simulink model "simulator"  (R2018b)
settings: Solver=VariableStepAuto  StartTime=0.0  StopTime=21  RelTol=1e-3  EnableMultiTasking=on
values from neighbouring files (symbols this model uses):
  acc_seed = randi(1000, [3, 1])    [init.m]
  anchors = [-4.715, -4.539, 2.67 ... (first row only)    [init.m]
  bias = [0.02998003, -0.03306038,  0.05456951 ... (first row only)    [init.m]
  gyro_seed = randi(1000, [3, 1])    [init.m]
  h = 0.002    [init.m]
  k = 2.2e-8    (= 2.2e-08)    [init_quadcopter_model.m]
  omega_max_lim = 2500    [init_inner_PD_d.m]
  omega_min_lim = 0    [init_inner_PD_d.m]
  outlier_seed = randi(1000, [4, 1])    [init.m]
  P_init = diag([10000,10000,1,0.0001,0.0001,0.0001,0.0001,0.0001,0.0001])    [init.m]
  PosD = 0.24    [init.m]
  PosI = 0    [init.m]
  PosP = 0.20    (= 0.2)    [init.m]
  procent_modifier = 1.96    [init.m]
  Q = diag([4.8366*h*h 4.8366*h*h 0.4530*h*h 4.8366*h 4.8366*h 0.4530*h 0.0083*h 0.0083*h 0.0547*h].^2)    [init.m]
  q_init = [1; 0; 0; 0]    [init.m]
  R = [R_alti R_uwb]    [init.m]
  Rotmat_init = eye(3)    [init.m]
  uwb_seed = randi(1000, [4, 1])    [init.m]
  uwb_var = 0.0625    [init.m]
  x_hat_init = [0; 0; 0; 0; 0; 0; 0; 0; 0]    [init.m]
  yaw_seed = randi(1000, 1)    [init.m]
undefined symbols (not defined in the file or in its folder): sigbuilder_block
libraries: commchan3 x17, simulink x2, dspinverses x1, dspmtrx3 x1
settings Model: Creator=Daniel  LastModifiedBy=sstroobants
settings DataIOCC: LimitDataPoints=on
settings OptimizationCC: LifeSpan=inf
settings DebuggingCC: AllowSymbolicDim=off  SFUnexpectedBacktrackingDiag=warning  SFNoUnconditionalDefaultTransitionDiag=warning  UnderSpecifiedDimensionMsg=warning
settings ModelReferenceCC: PropagateSignalLabelsOutOfModel=off
settings SFSimCC: SimUseLocalCustomCode=off
settings RTWCC: RTWUseLocalCustomCode=off
settings CodeAppCC: StateflowObjectComments=on
settings GRTTargetCC: TargetLangStandard=C89/C90 (ANSI)
settings ConfigComp: CovMetricSettings=dw  CovHtmlReporting=on  CovSaveCumulativeToWorkspaceVar=on  CovSaveSingleToWorkspaceVar=on  CovExternalEMLEnable=off

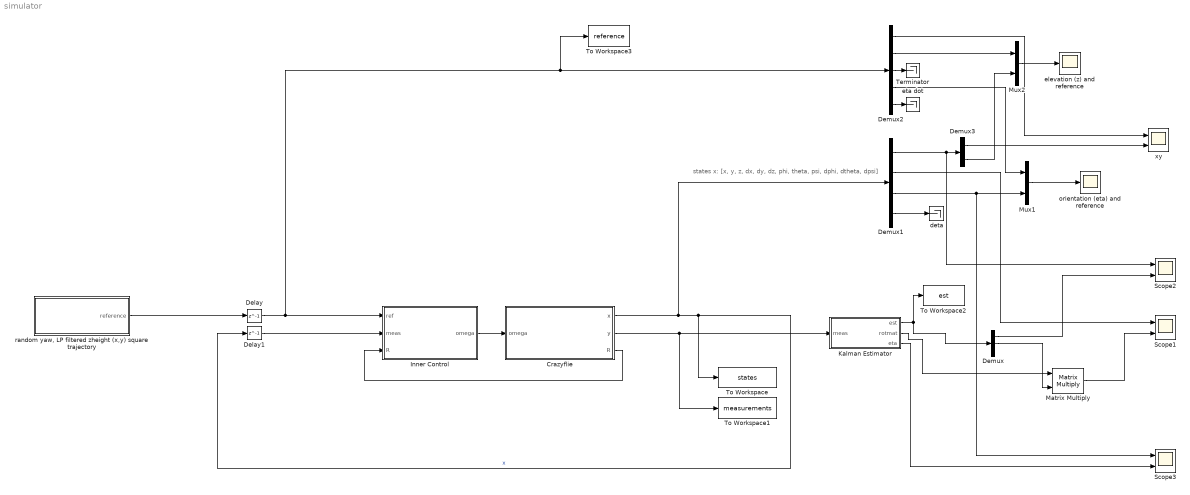
== system simulator ==
  note: states x: [x, y, z, dx, dy, dz, phi, theta, psi, dphi, dtheta, dpsi]
  "   deta" : Terminator
  "   eta dot" : Terminator
  Crazyflie : Subsystem
  Delay : Delay  DelayLength=1  InitialCondition=0  SampleTime=0.002
  Delay1 : Delay  DelayLength=1  InitialCondition=0  SampleTime=0.002
  Demux : Demux  Outputs=3
  Demux1 : Demux  Outputs=[3,3,3,3]
  Demux2 : Demux  Outputs=[2,1,3,3,3]
  Demux3 : Demux  Outputs=[2,1]
  Inner Control : Subsystem
  Kalman Estimator : Subsystem
  Matrix Multiply : Product  Multiplication=Matrix(*)
  Mux1 : Mux  Inputs=2
  Mux2 : Mux  Inputs=2
  Scope1 : Scope  NumInputPorts=2
  Scope2 : Scope  NumInputPorts=2
  Scope3 : Scope  NumInputPorts=2
  Terminator : Terminator
  To Workspace : ToWorkspace  VariableName=states  SaveFormat=Timeseries  SampleTime=-1
  To Workspace1 : ToWorkspace  VariableName=measurements  SaveFormat=Timeseries  SampleTime=-1
  To Workspace2 : ToWorkspace  VariableName=est  SaveFormat=Timeseries  SampleTime=-1
  To Workspace3 : ToWorkspace  VariableName=reference  SaveFormat=Timeseries  SampleTime=-1
  elevation (z) and reference : Scope
  orientation (eta) and reference : Scope
  "random yaw, LP filtered zheight (x,y) square trajectory " : Subsystem
  xy : Scope  NumInputPorts=2
  wires:
  Mux2/1 -> elevation (z) and reference/1
  Mux1/1 -> orientation (eta) and reference/1
  Demux2/5 -> "   eta dot"/1
  Demux2/1 -> xy/1
  Demux1/1 -> Demux3/1, Scope2/1
  Delay/1 -> To Workspace3/1, Demux2/1, Inner Control/1(ref)
  Delay1/1 -> Inner Control/2(meas)
  Demux1/4 -> "   deta"/1
  Demux3/1 -> xy/2
  "random yaw, LP filtered zheight (x,y) square trajectory "/1(reference) -> Delay/1
  Demux2/2 -> Mux2/1
  Demux3/2 -> Mux2/2
  Demux1/3 -> Scope3/1, Mux1/2
  Demux2/4 -> Mux1/1
  Inner Control/1(omega) -> Crazyflie/1(omega)
  Crazyflie/1(x) -> To Workspace/1, Delay1/1, Demux1/1  "x"
  Crazyflie/2(y) -> To Workspace1/1, Kalman Estimator/1(meas)
  Kalman Estimator/1(est) -> Demux/1, To Workspace2/1
  Demux/2 -> Matrix Multiply/2
  Demux1/2 -> Scope1/1
  Matrix Multiply/1 -> Scope1/2
  Kalman Estimator/2(rotmat) -> Matrix Multiply/1
  Demux/1 -> Scope2/2
  Kalman Estimator/3(eta) -> Scope3/2
  Crazyflie/3(R) -> Inner Control/3(R)
  Demux2/3 -> Terminator/1

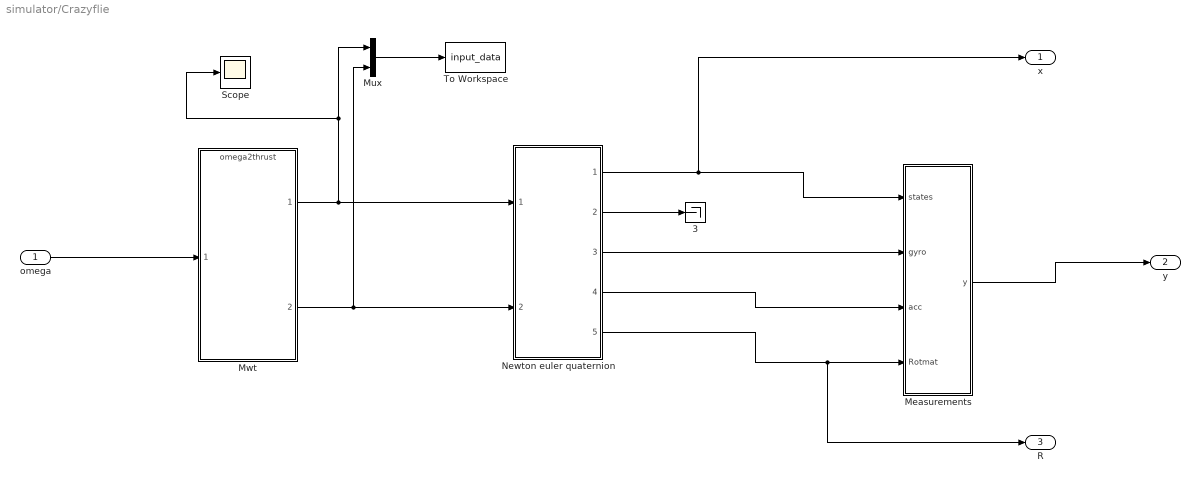
== system simulator/Crazyflie ==
  omega : Inport
  "   3" : Terminator
  Measurements : Subsystem
  Mux : Mux  Inputs=2
  Mwt : ModelReference  ModelNameDialog=omega2thrust.mdl  SimulationMode=Normal  ModelReferenceVersion=1.5
  Newton euler quaternion : ModelReference  ModelNameDialog=quadcopter_model_c_NewtonEuler.mdl  SimulationMode=Normal  ModelReferenceVersion=1.346
  Scope : Scope
  To Workspace : ToWorkspace  VariableName=input_data  SaveFormat=Timeseries  SampleTime=-1
  x : Outport
  y : Outport  Port=2
  R : Outport  Port=3
  wires:
  Newton euler quaternion/2 -> "   3"/1
  Newton euler quaternion/5 -> R/1, Measurements/4(Rotmat)
  Mwt/1 -> Mux/1, Scope/1, Newton euler quaternion/1
  omega/1 -> Mwt/1
  Newton euler quaternion/1 -> x/1, Measurements/1(states)
  Mwt/2 -> Mux/2, Newton euler quaternion/2
  Newton euler quaternion/3 -> Measurements/2(gyro)
  Newton euler quaternion/4 -> Measurements/3(acc)
  Measurements/1(y) -> y/1
  Mux/1 -> To Workspace/1

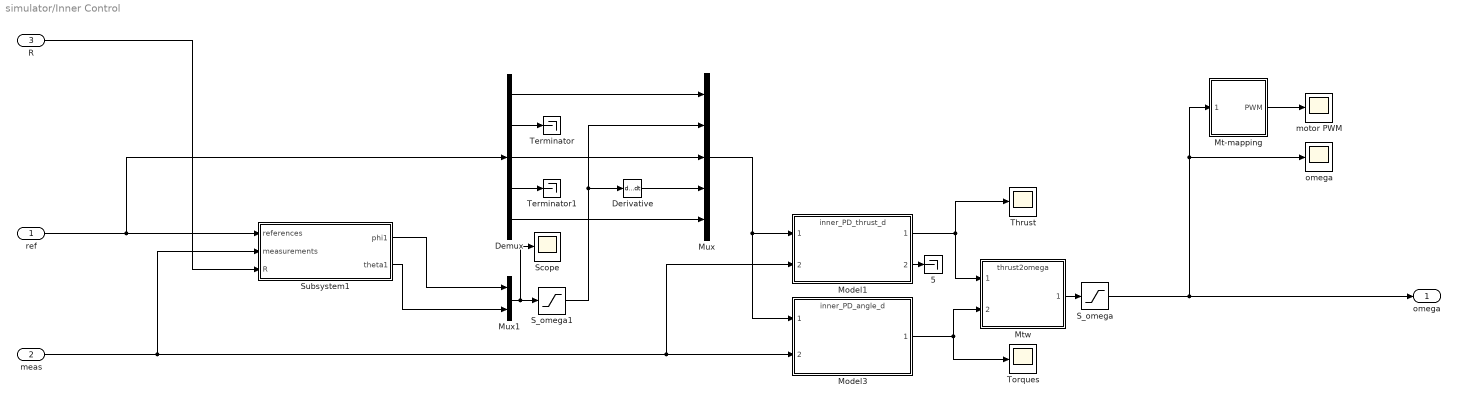
== system simulator/Inner Control ==
  ref : Inport
  meas : Inport  Port=2
  R : Inport  Port=3
  "   5" : Terminator
  Demux : Demux  Outputs=[6,2,1,2,1]
  Derivative : Derivative
  Model1 : ModelReference  ModelNameDialog=inner_PD_thrust_d.slx  SimulationMode=Normal  ModelReferenceVersion=1.83
  Model3 : ModelReference  ModelNameDialog=inner_PD_angle_d.slx  SimulationMode=Normal  ModelReferenceVersion=1.87
  Mt-mapping : Subsystem
  Mtw : ModelReference  ModelNameDialog=thrust2omega.mdl  SimulationMode=Normal  ModelReferenceVersion=1.5
  Mux : Mux  Inputs=[6,2,1,2,1]
  Mux1 : Mux  Inputs=2
  S_omega : Saturate  UpperLimit=omega_max_lim  LowerLimit=omega_min_lim
  S_omega1 : Saturate
  Scope : Scope
  Subsystem1 : Subsystem
  Terminator : Terminator
  Terminator1 : Terminator
  Thrust : Scope
  Torques : Scope
  motor PWM : Scope
  "omega " : Scope
  omega : Outport
  wires:
  Model1/2 -> "   5"/1
  Model3/1 -> Torques/1, Mtw/2
  Model1/1 -> Thrust/1, Mtw/1
  Mtw/1 -> S_omega/1
  S_omega/1 -> omega/1, Mt-mapping/1(omega), "omega "/1
  Mt-mapping/1(PWM) -> motor PWM/1
  ref/1 -> Subsystem1/1(references), Demux/1
  meas/1 -> Subsystem1/2(measurements), Model1/2, Model3/2
  Demux/1 -> Mux/1
  Mux1/1 -> Scope/1, S_omega1/1
  Derivative/1 -> Mux/4
  Demux/2 -> Terminator/1
  Demux/4 -> Terminator1/1
  Demux/3 -> Mux/3
  Demux/5 -> Mux/5
  Mux/1 -> Model3/1, Model1/1
  S_omega1/1 -> Derivative/1, Mux/2
  R/1 -> Subsystem1/3(R)
  Subsystem1/1(phi1) -> Mux1/1
  Subsystem1/2(theta1) -> Mux1/2

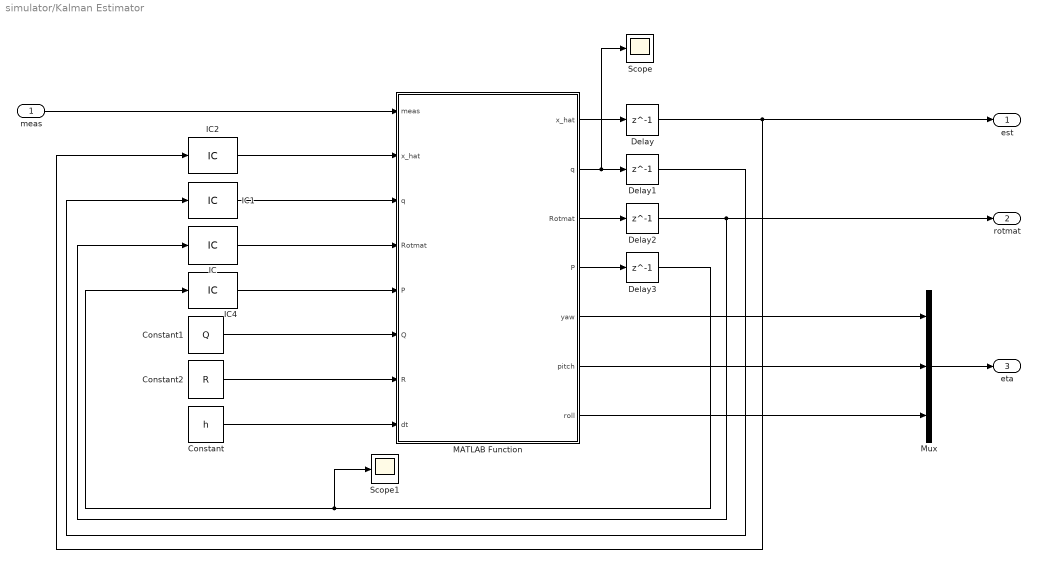
== system simulator/Kalman Estimator ==
  meas : Inport  PortDimensions=17
  Constant : Constant  Value=h
  Constant1 : Constant  Value=Q
  Constant2 : Constant  Value=R
  Delay{,1..3} (4 alike) : Delay  DelayLength=1
  IC : InitialCondition  Value=Rotmat_init
  IC1 : InitialCondition  Value=q_init
  IC2 : InitialCondition  Value=x_hat_init
  IC4 : InitialCondition  Value=P_init
  MATLAB Function : MATLAB Function  TreatAsAtomicUnit=on
  Mux : Mux  Inputs=3
  Scope : Scope
  Scope1 : Scope
  est : Outport  PortDimensions=9
  rotmat : Outport  Port=2  PortDimensions=[3 3]
  eta : Outport  Port=3  PortDimensions=3
  wires:
  meas/1 -> MATLAB Function/1(meas)
  Constant1/1 -> MATLAB Function/6(Q)
  IC/1 -> MATLAB Function/4("Rotmat ")
  IC1/1 -> MATLAB Function/3("q ")
  IC2/1 -> MATLAB Function/2("x_hat ")
  IC4/1 -> MATLAB Function/5("P ")
  MATLAB Function/1(x_hat) -> Delay/1
  MATLAB Function/2(q) -> Scope/1, Delay1/1
  MATLAB Function/3(Rotmat) -> Delay2/1
  MATLAB Function/4(P) -> Delay3/1
  Delay/1 -> est/1, IC2/1
  Delay1/1 -> IC1/1
  Delay2/1 -> IC/1, rotmat/1
  Delay3/1 -> Scope1/1, IC4/1
  Constant2/1 -> MATLAB Function/7(R)
  MATLAB Function/5(yaw) -> Mux/1
  MATLAB Function/6(pitch) -> Mux/2
  MATLAB Function/7(roll) -> Mux/3
  Mux/1 -> eta/1
  Constant/1 -> MATLAB Function/8(dt)

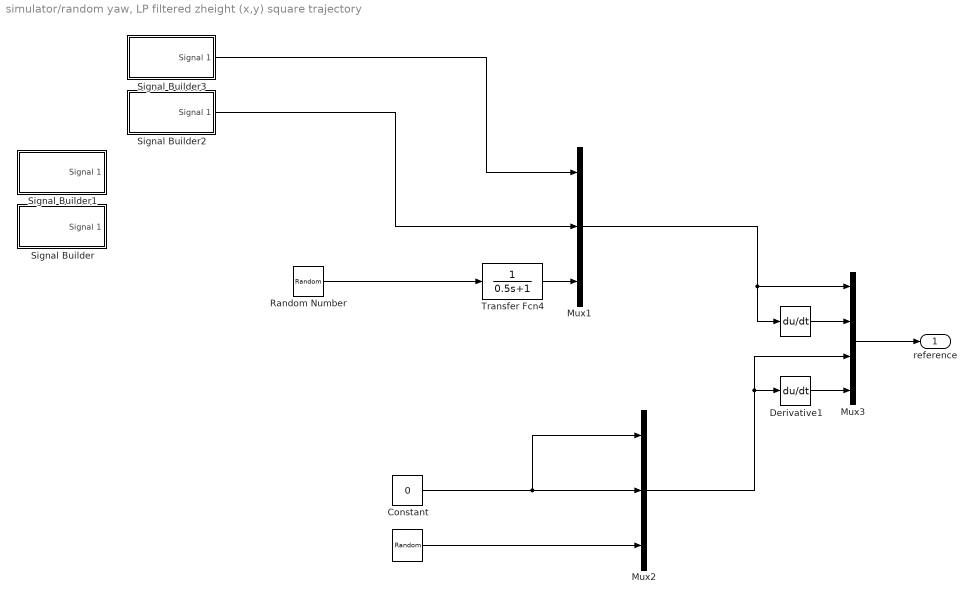
== system simulator/random yaw, LP filtered zheight (x,y) square trajectory  ==
  "   " : UniformRandomNumber  Minimum=-0.3  Maximum=0.3  Seed=yaw_seed  SampleTime=3
  "        " : Derivative
  Constant : Constant  Value=0
  Derivative1 : Derivative
  Mux1 : Mux  Inputs=3
  Mux2 : Mux  Inputs=3
  Mux3 : Mux  Inputs=[3,3,3,3]
  Random Number : RandomNumber  Mean=1.5  Variance=0.6  SampleTime=0.1
  Signal Builder : Subsystem  Tag=STV Subsys  LoadFcn=sigbuilder_block('load');  StartFcn=sigbuilder_block('start');  StopFcn=sigbuilder_block('stop');  ClipboardFcn=sigbuilder_block('clipboard');  mask(Sigbuilder block){tuvar=[0:10]}
      mask help: Simulink:masks:SigbuilderBlock_MD
      mask init:
      | if ~strcmp(get_param(bdroot(gcbh),'SimulationStatus'),'stopped') tuvar = sigbuilder_block('maskInit'); end
      settings: CopyFcn=sigbuilder_block('copy');  DeleteFcn=sigbuilder_block('delete');  ModelCloseFcn=sigbuilder_block('modelClose');  PreSaveFcn=sigbuilder_block('preSave');  PauseFcn=sigbuilder_block('pause');  ContinueFcn=sigbuilder_block('continue');  NameChangeFcn=sigbuilder_block('namechange');  OpenFcn=sigbuilder_block('open',[411 173.25 603 399.75 ]);  CloseFcn=sigbuilder_block('close');
      mask Display: plot(0, 0, 100, 100,[2, 2, 32, 32, 2], [68, 8, 8, 68, 68],[32, 2], [38, 38], [32, 19, 2],[53, 60, 44], [32, 17, 17, 2],[16, 16, 31, 31]);txt = getActiveGroup(gcbh);text(2, 100, txt,'verticalAlignment', 'top');
  Signal Builder1 : Subsystem  Tag=STV Subsys  LoadFcn=sigbuilder_block('load');  StartFcn=sigbuilder_block('start');  StopFcn=sigbuilder_block('stop');  ClipboardFcn=sigbuilder_block('clipboard');  mask(Sigbuilder block){tuvar=[0:10]}
      mask help: Simulink:masks:SigbuilderBlock_MD
      mask init:
      | if ~strcmp(get_param(bdroot(gcbh),'SimulationStatus'),'stopped') tuvar = sigbuilder_block('maskInit'); end
      settings: CopyFcn=sigbuilder_block('copy');  DeleteFcn=sigbuilder_block('delete');  ModelCloseFcn=sigbuilder_block('modelClose');  PreSaveFcn=sigbuilder_block('preSave');  PauseFcn=sigbuilder_block('pause');  ContinueFcn=sigbuilder_block('continue');  NameChangeFcn=sigbuilder_block('namechange');  OpenFcn=sigbuilder_block('open',[411 173.25 603 399.75 ]);  CloseFcn=sigbuilder_block('close');
      mask Display: plot(0, 0, 100, 100,[2, 2, 32, 32, 2], [68, 8, 8, 68, 68],[32, 2], [38, 38], [32, 19, 2],[53, 60, 44], [32, 17, 17, 2],[16, 16, 31, 31]);txt = getActiveGroup(gcbh);text(2, 100, txt,'verticalAlignment', 'top');
  Signal Builder2 : Subsystem  Tag=STV Subsys  LoadFcn=sigbuilder_block('load');  StartFcn=sigbuilder_block('start');  StopFcn=sigbuilder_block('stop');  ClipboardFcn=sigbuilder_block('clipboard');  mask(Sigbuilder block){tuvar=[0:10]}
      mask help: Simulink:masks:SigbuilderBlock_MD
      mask init:
      | if ~strcmp(get_param(bdroot(gcbh),'SimulationStatus'),'stopped') tuvar = sigbuilder_block('maskInit'); end
      settings: CopyFcn=sigbuilder_block('copy');  DeleteFcn=sigbuilder_block('delete');  ModelCloseFcn=sigbuilder_block('modelClose');  PreSaveFcn=sigbuilder_block('preSave');  PauseFcn=sigbuilder_block('pause');  ContinueFcn=sigbuilder_block('continue');  NameChangeFcn=sigbuilder_block('namechange');  OpenFcn=sigbuilder_block('open',[406.5 170.25 603 399.75 ]);  CloseFcn=sigbuilder_block('close');
      mask Display: plot(0, 0, 100, 100,[2, 2, 32, 32, 2], [68, 8, 8, 68, 68],[32, 2], [38, 38], [32, 19, 2],[53, 60, 44], [32, 17, 17, 2],[16, 16, 31, 31]);txt = getActiveGroup(gcbh);text(2, 100, txt,'verticalAlignment', 'top');
  Signal Builder3 : Subsystem  Tag=STV Subsys  LoadFcn=sigbuilder_block('load');  StartFcn=sigbuilder_block('start');  StopFcn=sigbuilder_block('stop');  ClipboardFcn=sigbuilder_block('clipboard');  mask(Sigbuilder block){tuvar=[0:10]}
      mask help: Simulink:masks:SigbuilderBlock_MD
      mask init:
      | if ~strcmp(get_param(bdroot(gcbh),'SimulationStatus'),'stopped') tuvar = sigbuilder_block('maskInit'); end
      settings: CopyFcn=sigbuilder_block('copy');  DeleteFcn=sigbuilder_block('delete');  ModelCloseFcn=sigbuilder_block('modelClose');  PreSaveFcn=sigbuilder_block('preSave');  PauseFcn=sigbuilder_block('pause');  ContinueFcn=sigbuilder_block('continue');  NameChangeFcn=sigbuilder_block('namechange');  OpenFcn=sigbuilder_block('open',[407.25 169.5 610.5 399.75 ]);  CloseFcn=sigbuilder_block('close');
      mask Display: plot(0, 0, 100, 100,[2, 2, 32, 32, 2], [68, 8, 8, 68, 68],[32, 2], [38, 38], [32, 19, 2],[53, 60, 44], [32, 17, 17, 2],[16, 16, 31, 31]);txt = getActiveGroup(gcbh);text(2, 100, txt,'verticalAlignment', 'top');
  Transfer Fcn4 : TransferFcn  Denominator=[0.5 1]
  reference : Outport
  wires:
  Mux3/1 -> reference/1
  Derivative1/1 -> Mux3/4
  "        "/1 -> Mux3/2
  Mux2/1 -> Mux3/3, Derivative1/1
  Constant/1 -> Mux2/1, Mux2/2
  Transfer Fcn4/1 -> Mux1/3
  Mux1/1 -> "        "/1, Mux3/1
  Random Number/1 -> Transfer Fcn4/1
  "   "/1 -> Mux2/3
  Signal Builder3/1(Signal 1) -> Mux1/1
  Signal Builder2/1(Signal 1) -> Mux1/2

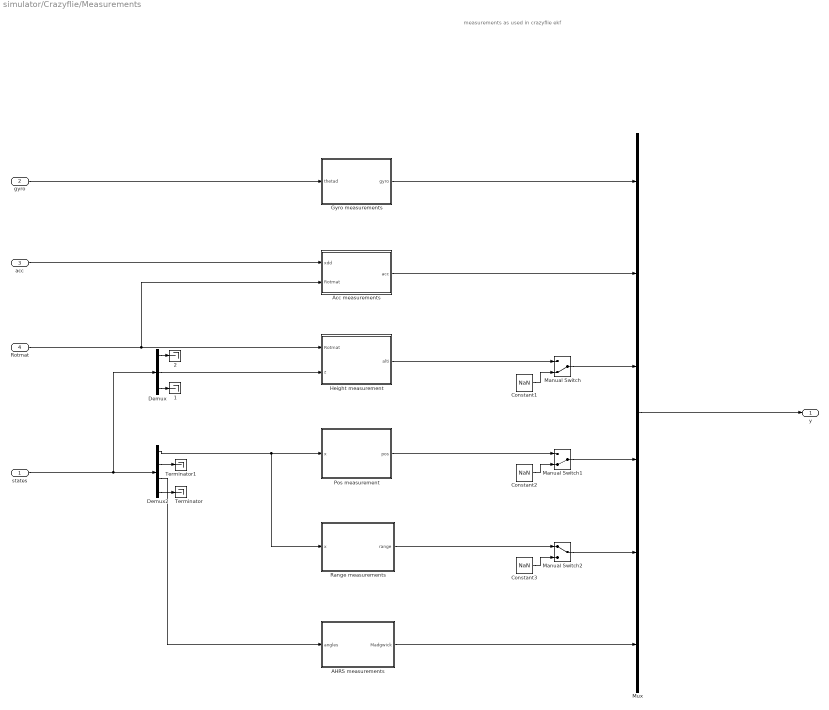
== system simulator/Crazyflie/Measurements ==
  note: measurements as used in crazyflie ekf
  states : Inport
  gyro : Inport  Port=2
  acc : Inport  Port=3
  Rotmat : Inport  Port=4
  "   1" : Terminator
  "   2" : Terminator
  AHRS measurements : Subsystem
  Acc measurements : Subsystem
  Constant1 : Constant  Value=NaN
  Constant2 : Constant  Value=NaN
  Constant3 : Constant  Value=NaN
  Demux : Demux  Outputs=[2 1 9]
  Demux2 : Demux  Outputs=[3 3 3 3]
  Gyro measurements : Subsystem
  Height measurement : Subsystem
  Manual Switch : ManualSwitch  CurrentSetting=0
  Manual Switch1 : ManualSwitch  CurrentSetting=0
  Manual Switch2 : ManualSwitch
  Mux : Mux  Inputs=[3 3 1 3 4 3]
  Pos measurement : Subsystem
  Range measurements : Subsystem
  Terminator : Terminator
  Terminator1 : Terminator
  y : Outport
  wires:
  Mux/1 -> y/1
  Demux/1 -> "   2"/1
  states/1 -> Demux/1, Demux2/1
  Demux2/1 -> Range measurements/1(x), Pos measurement/1(x)
  Demux/3 -> "   1"/1
  Constant1/1 -> Manual Switch/2
  Manual Switch/1 -> Mux/3
  Constant2/1 -> Manual Switch1/2
  Manual Switch1/1 -> Mux/4
  Manual Switch2/1 -> Mux/5
  Constant3/1 -> Manual Switch2/2
  Range measurements/1(range) -> Manual Switch2/1
  Rotmat/1 -> Acc measurements/2(Rotmat), Height measurement/1(Rotmat)
  gyro/1 -> Gyro measurements/1(thetad)
  Gyro measurements/1(gyro) -> Mux/1
  acc/1 -> Acc measurements/1(xdd)
  Acc measurements/1(acc) -> Mux/2
  Demux2/2 -> Terminator1/1
  Pos measurement/1(pos) -> Manual Switch1/1
  Demux/2 -> Height measurement/2(z)
  Height measurement/1(alti) -> Manual Switch/1
  Demux2/4 -> Terminator/1
  Demux2/3 -> AHRS measurements/1(angles)
  AHRS measurements/1(Madgwick) -> Mux/6

== system simulator/Inner Control/Mt-mapping ==
  omega : Inport
  Constant : Constant  Value=k
  MATLAB Function : MATLAB Function  TreatAsAtomicUnit=on
  PWM : Outport
  wires:
  MATLAB Function/1(PWM) -> PWM/1
  omega/1 -> MATLAB Function/1(omega)
  Constant/1 -> MATLAB Function/2(k)

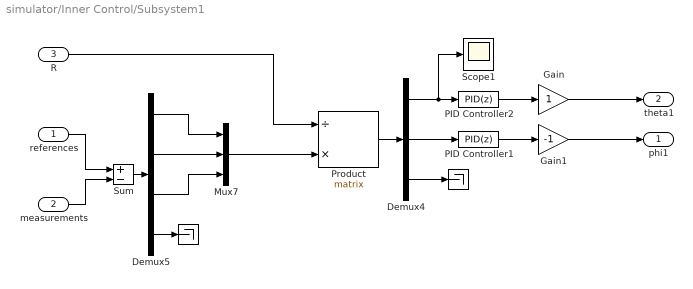
== system simulator/Inner Control/Subsystem1 ==
  references : Inport
  measurements : Inport  Port=2
  R : Inport  Port=3
  "      " : Terminator
  "       " : Terminator
  Demux4 : Demux  Outputs=[1,1,1]
  Demux5 : Demux  Outputs=[1,1,1,9]
  Gain : Gain
  Gain1 : Gain  Gain=-1
  Mux7 : Mux  Inputs=3
  PID Controller1 : simulink/Continuous/PID Controller  Controller=PID  Form=Parallel  TimeDomain=Discrete-time  SampleTime=-1  IntegratorMethod=Forward Euler  FilterMethod=Forward Euler  ControllerParametersSource=internal  P=PosP  I=PosI  D=PosD  UseFilter=on  N=100  TunerSelectOption=Transfer Function Based (PID Tuner App)  InitialConditionSource=internal  InitialConditionForIntegrator=0  InitialConditionForFilter=0  DifferentiatorICPrevScaledInput=0  ExternalReset=none  TrackingMode=off  Kt=1  LimitOutput=off  UpperSaturationLimit=inf  LowerSaturationLimit=-inf  LinearizeAsGain=on  AntiWindupMode=none  Kb=1  POutMin=[]  POutMax=[]  IOutMin=[]  IOutMax=[]  DOutMin=[]  DOutMax=[]  NOutMin=[]  NOutMax=[]  SumOutMin=[]  SumOutMax=[]  SaturationOutMin=[]  SaturationOutMax=[]  PParamMin=[]  PParamMax=[]  IParamMin=[]  IParamMax=[]  DParamMin=[]  DParamMax=[]  NParamMin=[]  NParamMax=[]  KbParamMin=[]  KbParamMax=[]  KtParamMin=[]  KtParamMax=[]  KbOutMin=[]  KbOutMax=[]  KtOutMin=[]  KtOutMax=[]  IntegratorOutMin=[]  IntegratorOutMax=[]  FilterOutMin=[]  FilterOutMax=[]  SumI1OutMin=[]  SumI1OutMax=[]  SumI2OutMin=[]  SumI2OutMax=[]  SumI3OutMin=[]  SumI3OutMax=[]  SumI4OutMin=[]  SumI4OutMax=[]  SumDOutMin=[]  SumDOutMax=[]  DifferentiatorOutMin=[]  DifferentiatorOutMax=[]  FilterDiffOutCoefMin=[]  FilterDiffOutCoefMax=[]  ReciprocalOutMin=[]  ReciprocalOutMax=[]  SumDenOutMin=[]  SumDenOutMax=[]  SumNumOutMin=[]  SumNumOutMax=[]  DivideOutMin=[]  DivideOutMax=[]  IntegratorContinuousStateAttributes=''  IntegratorStateMustResolveToSignalObject=off  IntegratorRTWStateStorageClass=Auto  FilterContinuousStateAttributes=''  FilterStateMustResolveToSignalObject=off  FilterRTWStateStorageClass=Auto  ParallelPVariant=InternalParameters  IdealPVariant=Disabled  IVariant=InternalParameters  DVariant=InternalParameters  IntegratorVariant=Discrete  SatVariant=Disabled  AWVariant=Passthrough  PCopyVariant=Disabled  TRVariant=Disabled  FdbkBlocksVariant=Forward  IdealPFdbkVariant=Disabled  SatFdbkVariant=Disabled  DerivativeFilterVariant=ForwardEulerFilter  NVariant=InternalParameters  NCopyVariant=Disabled  FilterICVariant=InternalICsFilter  IntegratorICVariant=InternalICs  ExternalResetVariant=Disabled  TRSumVariant=Passthrough  SumFdbkVariant=Disabled  SumVariant=Sum_PID
  PID Controller2 : simulink/Continuous/PID Controller  Controller=PID  Form=Parallel  TimeDomain=Discrete-time  SampleTime=-1  IntegratorMethod=Forward Euler  FilterMethod=Forward Euler  ControllerParametersSource=internal  P=PosP  I=PosI  D=PosD  UseFilter=on  N=100  TunerSelectOption=Transfer Function Based (PID Tuner App)  InitialConditionSource=internal  InitialConditionForIntegrator=0  InitialConditionForFilter=0  DifferentiatorICPrevScaledInput=0  ExternalReset=none  TrackingMode=off  Kt=1  LimitOutput=off  UpperSaturationLimit=inf  LowerSaturationLimit=-inf  LinearizeAsGain=on  AntiWindupMode=none  Kb=1  POutMin=[]  POutMax=[]  IOutMin=[]  IOutMax=[]  DOutMin=[]  DOutMax=[]  NOutMin=[]  NOutMax=[]  SumOutMin=[]  SumOutMax=[]  SaturationOutMin=[]  SaturationOutMax=[]  PParamMin=[]  PParamMax=[]  IParamMin=[]  IParamMax=[]  DParamMin=[]  DParamMax=[]  NParamMin=[]  NParamMax=[]  KbParamMin=[]  KbParamMax=[]  KtParamMin=[]  KtParamMax=[]  KbOutMin=[]  KbOutMax=[]  KtOutMin=[]  KtOutMax=[]  IntegratorOutMin=[]  IntegratorOutMax=[]  FilterOutMin=[]  FilterOutMax=[]  SumI1OutMin=[]  SumI1OutMax=[]  SumI2OutMin=[]  SumI2OutMax=[]  SumI3OutMin=[]  SumI3OutMax=[]  SumI4OutMin=[]  SumI4OutMax=[]  SumDOutMin=[]  SumDOutMax=[]  DifferentiatorOutMin=[]  DifferentiatorOutMax=[]  FilterDiffOutCoefMin=[]  FilterDiffOutCoefMax=[]  ReciprocalOutMin=[]  ReciprocalOutMax=[]  SumDenOutMin=[]  SumDenOutMax=[]  SumNumOutMin=[]  SumNumOutMax=[]  DivideOutMin=[]  DivideOutMax=[]  IntegratorContinuousStateAttributes=''  IntegratorStateMustResolveToSignalObject=off  IntegratorRTWStateStorageClass=Auto  FilterContinuousStateAttributes=''  FilterStateMustResolveToSignalObject=off  FilterRTWStateStorageClass=Auto  ParallelPVariant=InternalParameters  IdealPVariant=Disabled  IVariant=InternalParameters  DVariant=InternalParameters  IntegratorVariant=Discrete  SatVariant=Disabled  AWVariant=Passthrough  PCopyVariant=Disabled  TRVariant=Disabled  FdbkBlocksVariant=Forward  IdealPFdbkVariant=Disabled  SatFdbkVariant=Disabled  DerivativeFilterVariant=ForwardEulerFilter  NVariant=InternalParameters  NCopyVariant=Disabled  FilterICVariant=InternalICsFilter  IntegratorICVariant=InternalICs  ExternalResetVariant=Disabled  TRSumVariant=Passthrough  SumFdbkVariant=Disabled  SumVariant=Sum_PID
  Product : Product  Inputs=/*  Multiplication=Matrix(*)
  Scope1 : Scope
  Sum : Sum  Inputs=+-
  phi1 : Outport
  theta1 : Outport  Port=2
  wires:
  Sum/1 -> Demux5/1
  measurements/1 -> Sum/2
  Demux4/1 -> Scope1/1, PID Controller2/1
  Product/1 -> Demux4/1
  Demux5/2 -> Mux7/2
  Mux7/1 -> Product/2
  Gain1/1 -> phi1/1
  R/1 -> Product/1
  PID Controller2/1 -> Gain/1
  Demux5/4 -> "      "/1
  Demux4/3 -> "       "/1
  Demux5/1 -> Mux7/1
  references/1 -> Sum/1
  Gain/1 -> theta1/1
  PID Controller1/1 -> Gain1/1
  Demux5/3 -> Mux7/3
  Demux4/2 -> PID Controller1/1

== system simulator/random yaw, LP filtered zheight (x,y) square trajectory /Signal Builder ==
  Demux : Demux  Tag=STV Demux  Outputs=1
  FromWs : FromWorkspace  Tag=STV FromWs  VariableName=tuvar  SampleTime=0
      SigBuilderData=|
      | common.afterFinalStr = 'Extrapolate'
      | common.sampleTime = 0
      | dataSet.timeRange = [0 21]
      | dataSet.name = 'Group 1'
      | sbobj.Groups.Name = 'Group 1'
      | sbobj.Groups.Signals.Name = 'Signal 1'
      | sbobj.Groups.Signals.XData = [0 1 3 7 11 15 19 21]
      | sbobj.Groups.Signals.YData = [0 0 1.5 -1.5 -1.5 1.5 1.5 0]
      | sbobj.Groups.TimeRange = [0 21]
  Signal 1 : Outport  Tag=STV Outport
  wires:
  Demux/1 -> Signal 1/1
  FromWs/1 -> Demux/1

== system simulator/random yaw, LP filtered zheight (x,y) square trajectory /Signal Builder1 ==
  Demux : Demux  Tag=STV Demux  Outputs=1
  FromWs : FromWorkspace  Tag=STV FromWs  VariableName=tuvar  SampleTime=0
      SigBuilderData=|
      | common.afterFinalStr = 'Extrapolate'
      | common.sampleTime = 0
      | dataSet.timeRange = [0 21]
      | dataSet.name = 'Group 1'
      | sbobj.Groups.Name = 'Group 1'
      | sbobj.Groups.Signals.Name = 'Signal 1'
      | sbobj.Groups.Signals.XData = [0 1 3 7 11 15 19 21]
      | sbobj.Groups.Signals.YData = [0 0 1.5 1.5 -1.5 -1.5 1.5 1.5]
      | sbobj.Groups.TimeRange = [0 21]
  Signal 1 : Outport  Tag=STV Outport
  wires:
  Demux/1 -> Signal 1/1
  FromWs/1 -> Demux/1

== system simulator/random yaw, LP filtered zheight (x,y) square trajectory /Signal Builder2 ==
  Demux : Demux  Tag=STV Demux  Outputs=1
  FromWs : FromWorkspace  Tag=STV FromWs  VariableName=tuvar  SampleTime=0
      SigBuilderData=|
      | common.afterFinalStr = 'Extrapolate'
      | common.sampleTime = 0
      | dataSet.timeRange = [0 21]
      | dataSet.name = 'Group 1'
      | sbobj.Groups.Name = 'Group 1'
      | sbobj.Groups.Signals.Name = 'Signal 1'
      | sbobj.Groups.Signals.XData = [0 1 3 7 11 15 19 21]
      | sbobj.Groups.Signals.YData = [0 0 3 -3 -3 3 3 0]
      | sbobj.Groups.TimeRange = [0 21]
  Signal 1 : Outport  Tag=STV Outport
  wires:
  Demux/1 -> Signal 1/1
  FromWs/1 -> Demux/1

== system simulator/random yaw, LP filtered zheight (x,y) square trajectory /Signal Builder3 ==
  Demux : Demux  Tag=STV Demux  Outputs=1
  FromWs : FromWorkspace  Tag=STV FromWs  VariableName=tuvar  SampleTime=0
      SigBuilderData=|
      | common.afterFinalStr = 'Extrapolate'
      | common.sampleTime = 0
      | dataSet.timeRange = [0 21]
      | dataSet.name = 'Group 1'
      | sbobj.Groups.Name = 'Group 1'
      | sbobj.Groups.Signals.Name = 'Signal 1'
      | sbobj.Groups.Signals.XData = [0 1 3 7 11 15 19 21]
      | sbobj.Groups.Signals.YData = [0 0 3 3 -3 -3 3 3]
      | sbobj.Groups.TimeRange = [0 21]
  Signal 1 : Outport  Tag=STV Outport
  wires:
  Demux/1 -> Signal 1/1
  FromWs/1 -> Demux/1

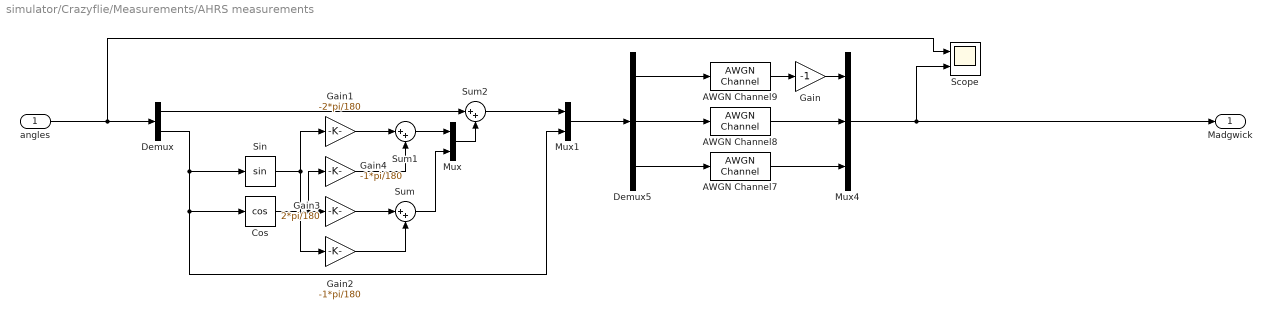
== system simulator/Crazyflie/Measurements/AHRS measurements ==
  angles : Inport
  AWGN Channel7 : commchan3/AWGN Channel  InputProcessing=Columns as channels (frame based)  seed=6784  noiseMode=Variance from mask  EbNodB=10  EsNodB=10  SNRdB=10  bitsPerSym=1  Ps=1  Tsym=1  variance=0.0000625
  AWGN Channel8 : commchan3/AWGN Channel  InputProcessing=Columns as channels (frame based)  seed=568658  noiseMode=Variance from mask  EbNodB=10  EsNodB=10  SNRdB=10  bitsPerSym=1  Ps=1  Tsym=1  variance=0.0000625
  AWGN Channel9 : commchan3/AWGN Channel  InputProcessing=Columns as channels (frame based)  seed=345  noiseMode=Variance from mask  EbNodB=10  EsNodB=10  SNRdB=10  bitsPerSym=1  Ps=1  Tsym=1  variance=0.0000625
  Cos : Trigonometry  Operator=cos
  Demux : Demux  Outputs=[2,1]
  Demux5 : Demux  Outputs=3
  Gain : Gain  Gain=-1
  Gain1 : Gain  Gain=-2*pi/180
  Gain2 : Gain  Gain=-1*pi/180
  Gain3 : Gain  Gain=2*pi/180
  Gain4 : Gain  Gain=-1*pi/180
  Mux : Mux  Inputs=2
  Mux1 : Mux  Inputs=[2,1]
  Mux4 : Mux  Inputs=3
  Scope : Scope  NumInputPorts=2
  Sin : Trigonometry
  Sum : Sum  Inputs=|++
  Sum1 : Sum  Inputs=|++
  Sum2 : Sum  Inputs=|++
  Madgwick : Outport
  wires:
  Demux5/1 -> AWGN Channel9/1
  AWGN Channel8/1 -> Mux4/2
  AWGN Channel9/1 -> Gain/1
  Demux5/2 -> AWGN Channel8/1
  AWGN Channel7/1 -> Mux4/3
  Mux4/1 -> Scope/2, Madgwick/1
  Demux5/3 -> AWGN Channel7/1
  angles/1 -> Scope/1, Demux/1
  Gain/1 -> Mux4/1
  Demux/2 -> Mux1/2, Cos/1, Sin/1
  Sin/1 -> Gain2/1, Gain1/1
  Cos/1 -> Gain4/1, Gain3/1
  Gain3/1 -> Sum/1
  Gain2/1 -> Sum/2
  Gain1/1 -> Sum1/1
  Gain4/1 -> Sum1/2
  Sum1/1 -> Mux/1
  Sum/1 -> Mux/2
  Mux/1 -> Sum2/2
  Demux/1 -> Sum2/1
  Sum2/1 -> Mux1/1
  Mux1/1 -> Demux5/1

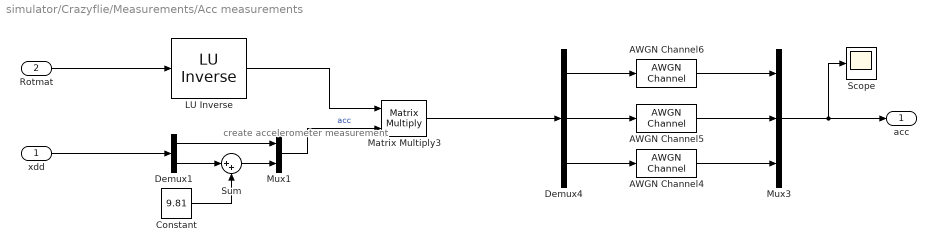
== system simulator/Crazyflie/Measurements/Acc measurements ==
  note: create accelerometer measurement
  xdd : Inport
  Rotmat : Inport  Port=2
  " LU Inverse" : dspinverses/ LU Inverse
      settings: SourceProductName=DSP System Toolbox
  AWGN Channel4 : commchan3/AWGN Channel  InputProcessing=Columns as channels (frame based)  seed=acc_seed(3)  noiseMode=Variance from mask  EbNodB=10  EsNodB=10  SNRdB=10  bitsPerSym=1  Ps=1  Tsym=1  variance=0.45
  AWGN Channel5 : commchan3/AWGN Channel  InputProcessing=Columns as channels (frame based)  seed=acc_seed(2)  noiseMode=Variance from mask  EbNodB=10  EsNodB=10  SNRdB=10  bitsPerSym=1  Ps=1  Tsym=1  variance=4.8
  AWGN Channel6 : commchan3/AWGN Channel  InputProcessing=Columns as channels (frame based)  seed=acc_seed(1)  noiseMode=Variance from mask  EbNodB=10  EsNodB=10  SNRdB=10  bitsPerSym=1  Ps=1  Tsym=1  variance=4.8
  Constant : Constant  Value=9.81
  Demux1 : Demux  Outputs=[2 1]
  Demux4 : Demux  Outputs=3
  Matrix Multiply3 : Product  Multiplication=Matrix(*)
  Mux1 : Mux  Inputs=[2 1]
  Mux3 : Mux  Inputs=3
  Scope : Scope
  Sum : Sum  Inputs=|++
  acc : Outport
  wires:
  AWGN Channel5/1 -> Mux3/2
  Constant/1 -> Sum/2
  AWGN Channel6/1 -> Mux3/1
  Mux1/1 -> Matrix Multiply3/2  "acc"
  Sum/1 -> Mux1/2
  Demux4/2 -> AWGN Channel5/1
  Demux4/3 -> AWGN Channel4/1
  Demux1/1 -> Mux1/1
  Demux4/1 -> AWGN Channel6/1
  Mux3/1 -> Scope/1, acc/1
  xdd/1 -> Demux1/1
  " LU Inverse"/1 -> Matrix Multiply3/1
  Demux1/2 -> Sum/1
  Matrix Multiply3/1 -> Demux4/1
  AWGN Channel4/1 -> Mux3/3
  Rotmat/1 -> " LU Inverse"/1

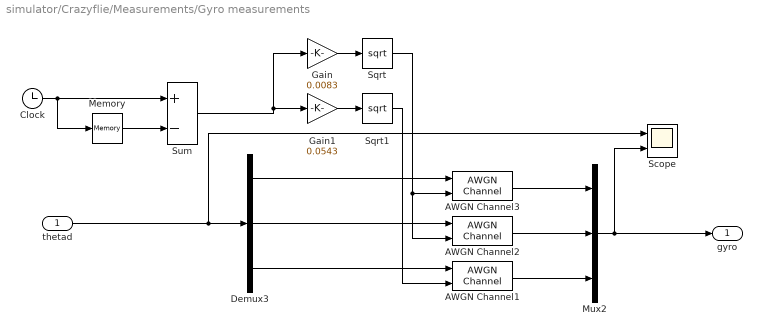
== system simulator/Crazyflie/Measurements/Gyro measurements ==
  thetad : Inport
  AWGN Channel1 : commchan3/AWGN Channel  InputProcessing=Columns as channels (frame based)  seed=gyro_seed(3)  noiseMode=Variance from port  EbNodB=10  EsNodB=10  SNRdB=10  bitsPerSym=1  Ps=1  Tsym=1  variance=0.00543
  AWGN Channel2 : commchan3/AWGN Channel  InputProcessing=Columns as channels (frame based)  seed=gyro_seed(2)  noiseMode=Variance from port  EbNodB=10  EsNodB=10  SNRdB=10  bitsPerSym=1  Ps=1  Tsym=1  variance=0.00083
  AWGN Channel3 : commchan3/AWGN Channel  InputProcessing=Columns as channels (frame based)  seed=gyro_seed(1)  noiseMode=Variance from port  EbNodB=10  EsNodB=10  SNRdB=10  bitsPerSym=1  Ps=1  Tsym=1  variance=0.0083
  Clock : Clock
  Demux3 : Demux  Outputs=3
  Gain : Gain  Gain=0.0083
  Gain1 : Gain  Gain=0.0543
  Memory : Memory
  Mux2 : Mux  Inputs=3
  Scope : Scope  NumInputPorts=2
  Sqrt : Sqrt  SaturateOnIntegerOverflow=on
  Sqrt1 : Sqrt  SaturateOnIntegerOverflow=on
  Sum : Sum  Inputs=+-
  gyro : Outport
  wires:
  AWGN Channel2/1 -> Mux2/2
  AWGN Channel3/1 -> Mux2/1
  Mux2/1 -> Scope/2, gyro/1
  thetad/1 -> Scope/1, Demux3/1
  Demux3/1 -> AWGN Channel3/1
  AWGN Channel1/1 -> Mux2/3
  Demux3/2 -> AWGN Channel2/1
  Demux3/3 -> AWGN Channel1/1
  Sum/1 -> Gain/1, Gain1/1
  Clock/1 -> Sum/1, Memory/1
  Memory/1 -> Sum/2
  Gain/1 -> Sqrt/1
  Gain1/1 -> Sqrt1/1
  Sqrt/1 -> AWGN Channel2/2, AWGN Channel3/2
  Sqrt1/1 -> AWGN Channel1/2

== system simulator/Crazyflie/Measurements/Height measurement ==
  note: create height measurement
  Rotmat : Inport
  z : Inport  Port=2
  AWGN Channel : commchan3/AWGN Channel  InputProcessing=Columns as channels (frame based)  seed=7  noiseMode=Variance from mask  EbNodB=10  EsNodB=10  SNRdB=10  bitsPerSym=1  Ps=1  Tsym=1  variance=0.0429
  Divide : Product  Inputs=*/
  Submatrix : dspmtrx3/Submatrix  RowSpan=One row  RowStartMode=Last  RowStartIndex=1  RowEndMode=Last  RowEndIndex=1  ColSpan=One column  ColStartMode=Last  ColStartIndex=1  ColEndMode=Last  ColEndIndex=1
  alti : Outport
  wires:
  Submatrix/1 -> Divide/2
  Divide/1 -> AWGN Channel/1  "alti"
  z/1 -> Divide/1
  AWGN Channel/1 -> alti/1
  Rotmat/1 -> Submatrix/1

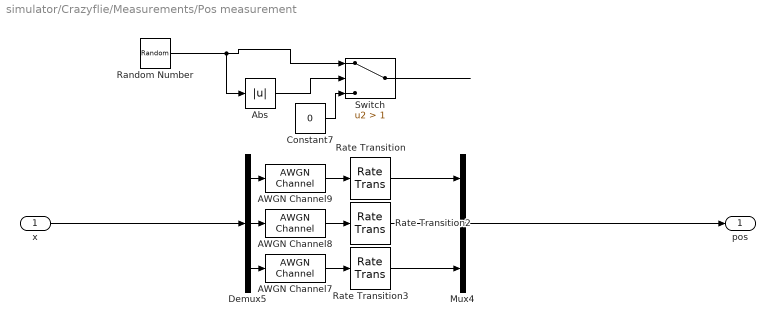
== system simulator/Crazyflie/Measurements/Pos measurement ==
  x : Inport
  AWGN Channel7 : commchan3/AWGN Channel  InputProcessing=Columns as channels (frame based)  seed=10  noiseMode=Variance from mask  EbNodB=10  EsNodB=10  SNRdB=10  bitsPerSym=1  Ps=1  Tsym=1  variance=0.0625
  AWGN Channel8 : commchan3/AWGN Channel  InputProcessing=Columns as channels (frame based)  seed=9  noiseMode=Variance from mask  EbNodB=10  EsNodB=10  SNRdB=10  bitsPerSym=1  Ps=1  Tsym=1  variance=0.0625
  AWGN Channel9 : commchan3/AWGN Channel  InputProcessing=Columns as channels (frame based)  seed=23340  noiseMode=Variance from mask  EbNodB=10  EsNodB=10  SNRdB=10  bitsPerSym=1  Ps=1  Tsym=1  variance=0.0625
  Abs : Abs
  Constant7 : Constant  Value=0
  Demux5 : Demux  Outputs=3
  Mux4 : Mux  Inputs=3
  Random Number : RandomNumber  Variance=0.35  Seed=326  SampleTime=0.05
  Rate Transition : RateTransition  OutPortSampleTime=0.05
  Rate Transition2 : RateTransition  OutPortSampleTime=0.05
  Rate Transition3 : RateTransition  OutPortSampleTime=0.05
  Switch : Switch  Criteria=u2 > Threshold  Threshold=1
  pos : Outport
  wires:
  AWGN Channel9/1 -> Rate Transition/1
  Rate Transition2/1 -> Mux4/2
  Demux5/1 -> AWGN Channel9/1
  Rate Transition3/1 -> Mux4/3
  AWGN Channel7/1 -> Rate Transition3/1
  Random Number/1 -> Switch/1, Abs/1
  x/1 -> Demux5/1
  Demux5/2 -> AWGN Channel8/1
  Mux4/1 -> pos/1
  Rate Transition/1 -> Mux4/1
  Switch/1 -> ?
  AWGN Channel8/1 -> Rate Transition2/1
  Abs/1 -> Switch/2
  Demux5/3 -> AWGN Channel7/1
  Constant7/1 -> Switch/3

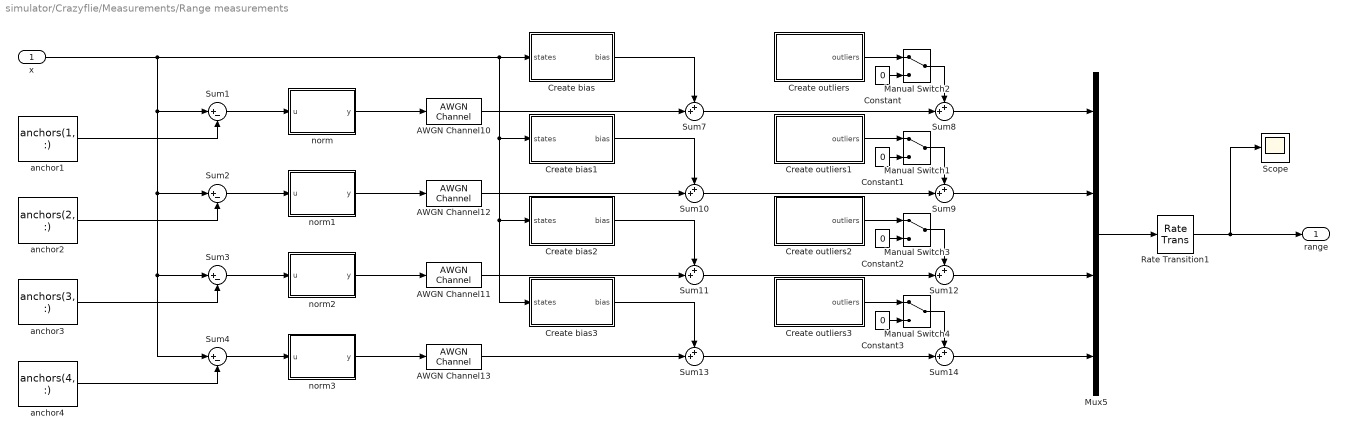
== system simulator/Crazyflie/Measurements/Range measurements ==
  x : Inport
  AWGN Channel10 : commchan3/AWGN Channel  InputProcessing=Columns as channels (frame based)  seed=uwb_seed(1)  noiseMode=Variance from mask  EbNodB=10  EsNodB=10  SNRdB=10  bitsPerSym=1  Ps=1  Tsym=1  variance=2*uwb_var*uwb_var
  AWGN Channel11 : commchan3/AWGN Channel  InputProcessing=Columns as channels (frame based)  seed=uwb_seed(3)  noiseMode=Variance from mask  EbNodB=10  EsNodB=10  SNRdB=10  bitsPerSym=1  Ps=1  Tsym=1  variance=2*uwb_var*uwb_var
  AWGN Channel12 : commchan3/AWGN Channel  InputProcessing=Columns as channels (frame based)  seed=uwb_seed(2)  noiseMode=Variance from mask  EbNodB=10  EsNodB=10  SNRdB=10  bitsPerSym=1  Ps=1  Tsym=1  variance=2*uwb_var*uwb_var
  AWGN Channel13 : commchan3/AWGN Channel  InputProcessing=Columns as channels (frame based)  seed=uwb_seed(4)  noiseMode=Variance from mask  EbNodB=10  EsNodB=10  SNRdB=10  bitsPerSym=1  Ps=1  Tsym=1  variance=2*uwb_var*uwb_var
  Constant{,1..3} (4 alike) : Constant  Value=0
  Create bias : Subsystem
  Create bias1 : Subsystem
  Create bias2 : Subsystem
  Create bias3 : Subsystem
  Create outliers : Subsystem
  Create outliers1 : Subsystem
  Create outliers2 : Subsystem
  Create outliers3 : Subsystem
  Manual Switch{1..4} (4 alike) : ManualSwitch
  Mux5 : Mux
  Rate Transition1 : RateTransition  OutPortSampleTime=0.04
  Scope : Scope
  Sum{1..4} (4 alike) : Sum  Inputs=|+-
  Sum{7..14} (8 alike) : Sum  Inputs=++|
  anchor1 : Constant  Value=anchors(1, :)
  anchor2 : Constant  Value=anchors(2, :)
  anchor3 : Constant  Value=anchors(3, :)
  anchor4 : Constant  Value=anchors(4, :)
  norm : MATLAB Function  TreatAsAtomicUnit=on
  norm1 : MATLAB Function  TreatAsAtomicUnit=on
  norm2 : MATLAB Function  TreatAsAtomicUnit=on
  norm3 : MATLAB Function  TreatAsAtomicUnit=on
  range : Outport  PortDimensions=4
  wires:
  Sum2/1 -> norm1/1(u)
  anchor3/1 -> Sum3/2
  Sum3/1 -> norm2/1(u)
  Sum1/1 -> norm/1(u)
  x/1 -> Sum4/1, Sum3/1, Sum2/1, Sum1/1, Create bias3/1(states), Create bias2/1(states), Create bias1/1(states), Create bias/1(states)
  Mux5/1 -> Rate Transition1/1
  Sum4/1 -> norm3/1(u)
  anchor4/1 -> Sum4/2
  anchor1/1 -> Sum1/2
  anchor2/1 -> Sum2/2
  Sum7/1 -> Sum8/2
  Sum10/1 -> Sum9/2
  Sum11/1 -> Sum12/2
  Sum13/1 -> Sum14/2
  Create outliers/1(outliers) -> Manual Switch2/1
  AWGN Channel13/1 -> Sum13/2
  norm3/1(y) -> AWGN Channel13/1
  AWGN Channel10/1 -> Sum7/2
  norm/1(y) -> AWGN Channel10/1
  norm1/1(y) -> AWGN Channel12/1
  norm2/1(y) -> AWGN Channel11/1
  AWGN Channel12/1 -> Sum10/2
  AWGN Channel11/1 -> Sum11/2
  Sum8/1 -> Mux5/1
  Sum9/1 -> Mux5/2
  Sum12/1 -> Mux5/3
  Sum14/1 -> Mux5/4
  Create bias/1(bias) -> Sum7/1
  Create bias3/1(bias) -> Sum13/1
  Create bias1/1(bias) -> Sum10/1
  Create bias2/1(bias) -> Sum11/1
  Rate Transition1/1 -> Scope/1, range/1
  Manual Switch2/1 -> Sum8/1
  Constant/1 -> Manual Switch2/2
  Manual Switch1/1 -> Sum9/1
  Constant1/1 -> Manual Switch1/2
  Create outliers1/1(outliers) -> Manual Switch1/1
  Manual Switch3/1 -> Sum12/1
  Constant2/1 -> Manual Switch3/2
  Create outliers2/1(outliers) -> Manual Switch3/1
  Manual Switch4/1 -> Sum14/1
  Constant3/1 -> Manual Switch4/2
  Create outliers3/1(outliers) -> Manual Switch4/1

== system simulator/Crazyflie/Measurements/Range measurements/Create bias ==
  states : Inport
  Constant : Constant  Value=bias(1, 3)
  Demux : Demux  Outputs=[1 1 1]
  Gain : Gain  Gain=bias(1, 1)
  Gain1 : Gain  Gain=bias(1, 2)
  Sum : Sum  Inputs=+|+|+
  Terminator : Terminator
  bias : Outport
  wires:
  Gain/1 -> Sum/1
  states/1 -> Demux/1
  Gain1/1 -> Sum/2
  Demux/2 -> Gain1/1
  Demux/3 -> Terminator/1
  Demux/1 -> Gain/1
  Sum/1 -> bias/1
  Constant/1 -> Sum/3

== system simulator/Crazyflie/Measurements/Range measurements/Create bias1 ==
  states : Inport
  Constant : Constant  Value=bias(2, 3)
  Demux : Demux  Outputs=[1 1 1]
  Gain : Gain  Gain=bias(2, 1)
  Gain1 : Gain  Gain=bias(2, 2)
  Sum : Sum  Inputs=+|+|+
  Terminator : Terminator
  bias : Outport
  wires:
  Gain/1 -> Sum/1
  states/1 -> Demux/1
  Gain1/1 -> Sum/2
  Demux/2 -> Gain1/1
  Demux/3 -> Terminator/1
  Demux/1 -> Gain/1
  Sum/1 -> bias/1
  Constant/1 -> Sum/3

== system simulator/Crazyflie/Measurements/Range measurements/Create bias2 ==
  states : Inport
  Constant : Constant  Value=bias(3, 3)
  Demux : Demux  Outputs=[1 1 1]
  Gain : Gain  Gain=bias(3, 1)
  Gain1 : Gain  Gain=bias(3, 2)
  Sum : Sum  Inputs=+|+|+
  Terminator : Terminator
  bias : Outport
  wires:
  Gain/1 -> Sum/1
  states/1 -> Demux/1
  Gain1/1 -> Sum/2
  Demux/2 -> Gain1/1
  Demux/3 -> Terminator/1
  Demux/1 -> Gain/1
  Sum/1 -> bias/1
  Constant/1 -> Sum/3

== system simulator/Crazyflie/Measurements/Range measurements/Create bias3 ==
  states : Inport
  Constant : Constant  Value=bias(4, 3)
  Demux : Demux  Outputs=[1 1 1]
  Gain : Gain  Gain=bias(4, 1)
  Gain1 : Gain  Gain=bias(4, 2)
  Sum : Sum  Inputs=+|+|+
  Terminator : Terminator
  bias : Outport
  wires:
  Gain/1 -> Sum/1
  states/1 -> Demux/1
  Gain1/1 -> Sum/2
  Demux/2 -> Gain1/1
  Demux/3 -> Terminator/1
  Demux/1 -> Gain/1
  Sum/1 -> bias/1
  Constant/1 -> Sum/3

== system simulator/Crazyflie/Measurements/Range measurements/Create outliers ==
  Abs : Abs
  Abs1 : Abs
  Constant : Constant  Value=1.5
  Constant7 : Constant  Value=0
  Gain : Gain  Gain=1/procent_modifier
  Random Number3 : RandomNumber  Seed=outlier_seed(1)  SampleTime=0.05
  Scope : Scope
  Switch : Switch  Criteria=u2 > Threshold  Threshold=procent_modifier
  Switch1 : Switch  Criteria=u2 > Threshold  Threshold=1.5
  outliers : Outport
  wires:
  Random Number3/1 -> Switch/1, Abs/1
  Abs/1 -> Switch/2
  Constant7/1 -> Switch/3
  Switch/1 -> Gain/1
  Gain/1 -> Switch1/3, Abs1/1
  Switch1/1 -> outliers/1, Scope/1
  Abs1/1 -> Switch1/2
  Constant/1 -> Switch1/1

== system simulator/Crazyflie/Measurements/Range measurements/Create outliers1 ==
  Abs : Abs
  Abs1 : Abs
  Constant : Constant  Value=1.5
  Constant7 : Constant  Value=0
  Gain : Gain  Gain=1/procent_modifier
  Random Number3 : RandomNumber  Seed=outlier_seed(2)  SampleTime=0.05
  Scope : Scope
  Switch : Switch  Criteria=u2 > Threshold  Threshold=procent_modifier
  Switch1 : Switch  Criteria=u2 > Threshold  Threshold=1.5
  outliers : Outport
  wires:
  Switch/1 -> Gain/1
  Switch1/1 -> outliers/1, Scope/1
  Abs1/1 -> Switch1/2
  Abs/1 -> Switch/2
  Constant/1 -> Switch1/1
  Random Number3/1 -> Switch/1, Abs/1
  Gain/1 -> Switch1/3, Abs1/1
  Constant7/1 -> Switch/3

== system simulator/Crazyflie/Measurements/Range measurements/Create outliers2 ==
  Abs : Abs
  Abs1 : Abs
  Constant : Constant  Value=1.5
  Constant7 : Constant  Value=0
  Gain : Gain  Gain=1/procent_modifier
  Random Number3 : RandomNumber  Seed=outlier_seed(3)  SampleTime=0.05
  Scope : Scope
  Switch : Switch  Criteria=u2 > Threshold  Threshold=procent_modifier
  Switch1 : Switch  Criteria=u2 > Threshold  Threshold=1.5
  outliers : Outport
  wires:
  Switch/1 -> Gain/1
  Switch1/1 -> outliers/1, Scope/1
  Abs1/1 -> Switch1/2
  Abs/1 -> Switch/2
  Constant/1 -> Switch1/1
  Random Number3/1 -> Switch/1, Abs/1
  Gain/1 -> Switch1/3, Abs1/1
  Constant7/1 -> Switch/3

== system simulator/Crazyflie/Measurements/Range measurements/Create outliers3 ==
  Abs : Abs
  Abs1 : Abs
  Constant : Constant  Value=1.5
  Constant7 : Constant  Value=0
  Gain : Gain  Gain=1/procent_modifier
  Random Number3 : RandomNumber  Seed=outlier_seed(4)  SampleTime=0.05
  Scope : Scope
  Switch : Switch  Criteria=u2 > Threshold  Threshold=procent_modifier
  Switch1 : Switch  Criteria=u2 > Threshold  Threshold=1.5
  outliers : Outport
  wires:
  Switch/1 -> Gain/1
  Switch1/1 -> outliers/1, Scope/1
  Abs1/1 -> Switch1/2
  Abs/1 -> Switch/2
  Constant/1 -> Switch1/1
  Random Number3/1 -> Switch/1, Abs/1
  Gain/1 -> Switch1/3, Abs1/1
  Constant7/1 -> Switch/3

== matlab function simulator/Crazyflie/Measurements/Range measurements/norm ==
  data: u input; y output
function y = fcn(u)

y = norm(u);

== matlab function simulator/Kalman Estimator/MATLAB Function ==
  data: meas input; x_hat input; x_hat output; q input; Rotmat input; P input; Q input; R input; q output; Rotmat output; P output; dt input; yaw output; pitch output; roll output
function [x_hat, q, Rotmat, P, yaw, pitch, roll] = EKF_crazyflie(meas, x_hat, q, Rotmat, P, Q, R, dt)

stateNum = 9;
dt2 = dt*dt;

w = meas(1:3);
if (all(abs(w) < 0.00001))
    w = w + 0.00001;
end
acc = meas(4:6)';
alti = meas(7);
uwb = meas(8:10);
uwb_range = meas(11:14);

R_alti = 0.0429;
R_uwb = 0.0625;

A = eye(stateNum);
e3 = [0;0;1];

w1_2t = w*dt/2;

% Calculate the Jacobian
A(1:3,1:3) = eye(3); A(1:3,4:6) = Rotmat*dt; A(1:3,7:9) = -Rotmat*matCrossPro(x_hat(4:6))*dt;
A(4:6,4:6) = eye(3)-matCrossPro(w)*dt;   A(4:6,7:9) = -9.81*matCrossPro(Rotmat'*e3)*dt;
A(7:9,7:9) = eye(3)+matCrossPro(-w1_2t)+(matCrossPro(-w1_2t))^2/2;

% Calculate state prediction based on forward euler
x_hat(1:3)=x_hat(1:3)+Rotmat*x_hat(4:6)*dt+Rotmat*acc'*dt2/2-9.81*e3*dt2/2;
x_hat(4:6)=x_hat(4:6)+acc'*dt-matCrossPro(w)*x_hat(4:6)*dt-9.81*Rotmat'*e3*dt;     

% Quadrotor z value cannot be less than zero..
if x_hat(3)<0
    x_hat(3)=0;x_hat(4)=0;x_hat(5)=0;x_hat(6)=0;
end

dq = angle2q(w*dt)';  q = quat_multiply(q,dq); q = q/norm(q);

% Calculate the covariance prediction
P = A*P*A' + Q;

if alti < 10 && ~isnan(alti)
    % ??Trying to prevent singularities??
    % Scalar Kalman update
    if Rotmat(3,3)>0.1
        predictD = x_hat(3)/Rotmat(3,3);
        measureD = alti;
        H = [0 0 1/Rotmat(3,3) 0 0 0 0 0 0];
        err = measureD-predictD;
        R = R_alti^2;
        K = P*H'/(H*P*H'+R);
        x_hat = x_hat+K*err;
        P = (eye(stateNum)-K*H)*P*(eye(stateNum)-K*H)'+K*R*K';
    end
end   

if ~isnan(uwb)
    for j=1:3
        predictD = x_hat(j);
        measureD = uwb(j);
        H = [0 0 0 0 0 0 0 0 0];
        H(j) = 1;
        err = measureD-predictD;
        R = R_uwb^2;
        K = P*H'/(H*P*H'+R);
        x_hat = x_hat+K*err;
        P = (eye(stateNum)-K*H)*P*(eye(stateNum)-K*H)'+K*R*K';
    end
end

if ~isnan(uwb_range)
    uwb_anchors = [-5 -5 0; -5 5 1.6; 5 5 1.6; 5 -5 2.7];
    for i = 1:4
        distXYZ = x_hat(1:3) - uwb_anchors(i, :)';
        predictD = norm(distXYZ);
        measureD = uwb_range(i);
        if abs(predictD) > 0.001
            H = [distXYZ(1)/predictD distXYZ(2)/predictD distXYZ(3)/predictD 0 0 0 0 0 0];
        else
            H = [1 0 0 0 0 0 0 0 0];
        end
        err = measureD-predictD;
        R = R_uwb^2;
        K = P*H'/(H*P*H'+R);
        x_hat = x_hat+K*err;
        P = (eye(stateNum)-K*H)*P*(eye(stateNum)-K*H)'+K*R*K';
    end
end

x_hat(7)=0;x_hat(8)=0;x_hat(9)=0;

tempq = zeros(4,1);
if ((abs(x_hat(7))>0.0001)||(abs(x_hat(8))>0.0001)||(abs(x_hat(9))>0.0001)) && ((abs(x_hat(7)) < 10) && (abs(x_hat(8)) < 10) && (abs(x_hat(9)) < 10))
    tempq=angle2q(x_hat(7:9));
    tempq=quat_multiply(q,tempq);
    q=tempq/norm(tempq);
    A=eye(stateNum);
    A(7:9,7:9)=A(7:9,7:9)+matCrossPro(-x_hat(7:9))/2+(matCrossPro(-x_hat(7:9)))^2/2;
    P = A*P*A';
end

Rotmat=quat2rotm(q');
x_hat(7)=0;x_hat(8)=0;x_hat(9)=0;

% for j=1:3
%     if (x_hat(j)<-100)
%         x_hat(j)=-100;
%     elseif (x_hat(j)>100)
%         x_hat(j)=100;
%     end
%     if (x_hat(3+j)<-10)
%         x_hat(3+j)=-10;
%     elseif (x_hat(j+3)>10)
%         x_hat(j+3)=10;
%     end
% end   
yaw  = atan2(2*(q(2)*q(3)+q(1)*q(4)) , q(1)*q(1) + q(2)*q(2) - q(3)*q(3) - q(4)*q(4));
pitch= asin(-2*(q(2)*q(4) - q(1)*q(3)));
roll = atan2(2*(q(3)*q(4)+q(1)*q(2)) , q(1)*q(1) - q(2)*q(2) - q(3)*q(3) + q(4)*q(4));

== matlab function simulator/Inner Control/Mt-mapping/MATLAB Function ==
  data: omega input; PWM output; k input
function PWM = Mt(omega, k)
%#codegen
rotor_thrusts = k.*omega.^2;
beta1 = 0.0877;
beta2 = 0.0660;
PWM =  -beta1/(2*beta2) + sqrt((beta1/(2*beta2))^2 + rotor_thrusts/beta2);

== matlab function simulator/Crazyflie/Measurements/Range measurements/norm1 ==
  data: u input; y output
function y = fcn(u)

y = norm(u);

== matlab function simulator/Crazyflie/Measurements/Range measurements/norm2 ==
  data: u input; y output
function y = fcn(u)

y = norm(u);

== matlab function simulator/Crazyflie/Measurements/Range measurements/norm3 ==
  data: u input; y output
function y = fcn(u)

y = norm(u);
